simulink model "quadrotor_control_template_R2018a"  (R2021a)
settings: Solver=VariableStepAuto  StartTime=0.0  StopTime=30  MaxStep=0.001  RelTol=1e-6
PreLoadFcn:
  | % first load parameters
  | initializeQuadrotorModel;
values from neighbouring files (symbols this model uses):
  xd0 = [1,2,5]+randn(1,3)    [Project.m]
undefined symbols (not defined in the file or in its folder): quadrotor, simPar
libraries: simulink x4, sharedtransform x1
settings Model: Creator=beniamino  LastModifiedBy=pasqu
settings SolverCC: ZeroCrossAlgorithm=Adaptive  AlgebraicLoopSolver=TrustRegion
settings DebuggingCC: IgnoredZcDiagnostic=none  ArithmeticOperatorsInVariantConditions=warning
settings SFSimCC: CustomCodeUndefinedFunction=UseInterfaceOnly

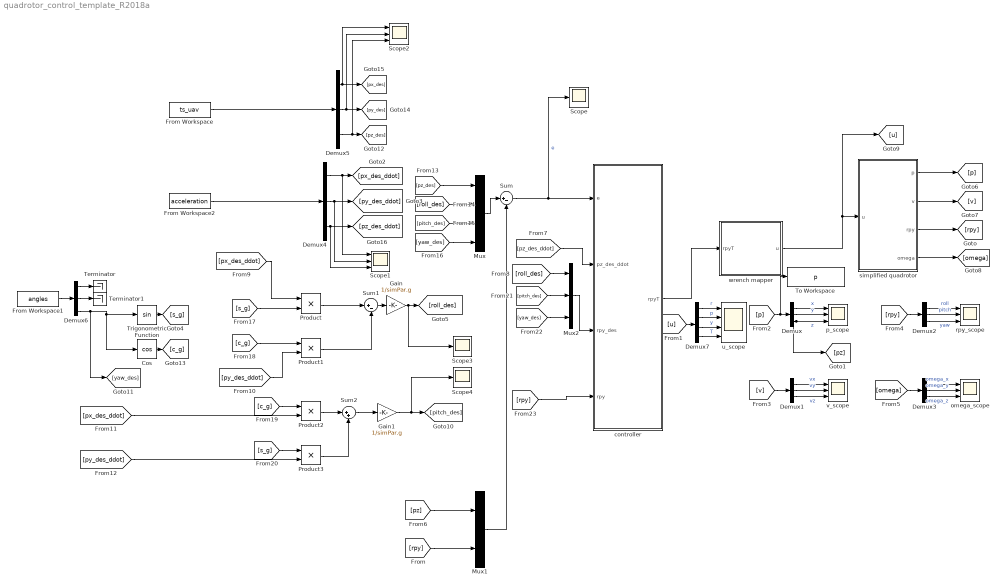
== system quadrotor_control_template_R2018a ==
  Cos : Trigonometry  Operator=cos
  Demux{,1..6} (7 alike) : Demux  Outputs=3
  Demux7 : Demux
  From Workspace : FromWorkspace  VariableName=ts_uav  SampleTime=-1
  From Workspace1 : FromWorkspace  VariableName=angles  SampleTime=-1  OutputAfterFinalValue=Holding final value
  From Workspace2 : FromWorkspace  VariableName=acceleration  SampleTime=-1
  Gain : Gain  Gain=1/simPar.g
  Gain1 : Gain  Gain=1/simPar.g
  Mux : Mux
  Mux1 : Mux  Inputs=2
  Mux2 : Mux  Inputs=3
  Product{,1..3} (4 alike) : Product
  Scope : Scope
  Scope1 : Scope  NumInputPorts=3
  Scope2 : Scope  NumInputPorts=3
  Scope3 : Scope
  Scope4 : Scope
  Sum : Sum  Inputs=|+-
  Sum1 : Sum  Inputs=|+-
  Sum2 : Sum  Inputs=|++
  Terminator : Terminator
  Terminator1 : Terminator
  To Workspace : ToWorkspace  VariableName=p  SaveFormat=Structure With Time  SampleTime=-1
  Trigonometric Function : Trigonometry
  controller : Subsystem
  omega_scope : Scope  NumInputPorts=3
  p_scope : Scope  NumInputPorts=3
  rpy_scope : Scope  NumInputPorts=3
  simplified quadrotor : Subsystem  mask(quadrotor model){F=quadrotor.mixer.F, M=quadrotor.mixer.M, mass=quadrotor.geometry.mass, gravity=simPar.g, inertia=quadrotor.geometry.I, maxRotorSpeed2=quadrotor.rotor.maxRotVelocity.^2, minRotorSpeed2=0, v_0=[0 0 0], omega_0=[0 0 0], ang_0=[0 0 0], p_0=xd0}
      mask prompts: F "F matrix"; M "M matrix"; mass "quadrotor mass"; inertia "inertia matrix"; maxRotorSpeed2 "Rotor max speed square"; minRotorSpeed2 "Rotor min speed square"; v_0 "initial linear velocity"; omega_0 "initial angular velocity"; ang_0 "initial angle"; p_0 "initial position"
      mask help: small angle simplified quadrotor model
      mask TypeOptions F: u2F/Gain
      mask TypeOptions M: u2M/Gain
      mask TypeOptions mass: mass/Value
      mask TypeOptions gravity: small angles rigid body dynamics/gravity/Value
      mask TypeOptions inertia: inertia/Value
      mask TypeOptions maxRotorSpeed2: saturate input/UpperLimit
      mask TypeOptions minRotorSpeed2: saturate input/LowerLimit
      mask TypeOptions v_0: small angles rigid body dynamics/ddp2dp/InitialCondition
      mask TypeOptions omega_0: small angles rigid body dynamics/domega2omega/InitialCondition
      mask TypeOptions ang_0: small angles rigid body dynamics/omega2ang/InitialCondition
      mask TypeOptions p_0: small angles rigid body dynamics/dp2p/InitialCondition
      mask DialogControl InitialConditionsGroupVar Prompt: Initial conditions
  u_scope : Scope  NumInputPorts=4
  v_scope : Scope  NumInputPorts=3
  wrench mapper : Subsystem  mask(wrench mapper){mapperMatrix=quadrotor.mixer.wrenchMapper}
      mask prompts: mapperMatrix "mapper matrix"
      mask help:
      | maps desired roll, pitch, yaw torque and total common thrust into the input vector u for a quadrotor.
      | input: [tau_roll, tau_pitch, tau_yaw, thrust]
      | input unit: [Nm, Nm, Nm, N]
      | output [u_1, u_2, u_3, u_3]
      | output unit: [rad^2/s^2]
      mask TypeOptions mapperMatrix: mapper/Gain
  wires:
  wrench mapper/1(u) -> [u], simplified quadrotor/1(u)
  simplified quadrotor/3(rpy) -> [rpy]
  simplified quadrotor/1(p) -> [p]
  simplified quadrotor/2(v) -> [v]
  simplified quadrotor/4(omega) -> [omega]
  Sum/1 -> Scope/1, controller/1(e)  "e"
  controller/1(rpyT) -> wrench mapper/1(rpyT)
  [p] -> To Workspace/1, Demux/1
  Demux/1 -> p_scope/1  "x"
  Demux/2 -> p_scope/2  "y"
  Demux/3 -> p_scope/3, [pz]  "z"
  [v] -> Demux1/1
  Demux1/2 -> v_scope/2  "vy"
  Demux1/3 -> v_scope/3  "vz"
  Demux1/1 -> v_scope/1  "vx"
  [rpy] -> Demux2/1
  Demux2/2 -> rpy_scope/2  "pitch"
  Demux2/3 -> rpy_scope/3  "yaw"
  Demux2/1 -> rpy_scope/1  "roll"
  [omega] -> Demux3/1
  Demux3/2 -> omega_scope/2  "omega_y"
  Demux3/3 -> omega_scope/3  "omega_z"
  Demux3/1 -> omega_scope/1  "omega_x"
  Mux/1 -> Sum/1
  [rpy] -> Mux1/2
  [pz] -> Mux1/1
  Mux1/1 -> Sum/2
  [pz_des_ddot] -> controller/2(pz_des_ddot)
  Mux2/1 -> controller/3(rpy_des)
  Demux4/1 -> Scope1/1, [px_des_ddot]
  Demux4/2 -> Scope1/2, [py_des_ddot]
  Demux4/3 -> Scope1/3, [pz_des_ddot]
  [px_des_ddot] -> Product/1
  [py_des_ddot] -> Product1/2
  Product/1 -> Sum1/1
  Product1/1 -> Sum1/2
  Sum1/1 -> Gain/1
  Gain/1 -> Scope3/1, [roll_des]
  [px_des_ddot] -> Product2/2
  [py_des_ddot] -> Product3/2
  Product2/1 -> Sum2/1
  Product3/1 -> Sum2/2
  Sum2/1 -> Gain1/1
  Gain1/1 -> Scope4/1, [pitch_des]
  Demux5/3 -> Scope2/3, [pz_des]
  Demux5/2 -> Scope2/2, [py_des]
  Demux5/1 -> Scope2/1, [px_des]
  [roll_des] -> Mux/2
  [pitch_des] -> Mux/3
  [yaw_des] -> Mux/4
  Trigonometric Function/1 -> [s_g]
  Cos/1 -> [c_g]
  [s_g] -> Product/2
  [c_g] -> Product1/1
  [c_g] -> Product2/1
  [s_g] -> Product3/1
  [pz_des] -> Mux/1
  [roll_des] -> Mux2/1
  [pitch_des] -> Mux2/2
  [yaw_des] -> Mux2/3
  [rpy] -> controller/4(rpy)
  From Workspace1/1 -> Demux6/1
  Demux6/3 -> Cos/1, Trigonometric Function/1, [yaw_des]
  Demux6/1 -> Terminator/1
  Demux6/2 -> Terminator1/1
  From Workspace/1 -> Demux5/1
  [u] -> Demux7/1
  Demux7/1 -> u_scope/1  "r"
  Demux7/2 -> u_scope/2  "p"
  Demux7/3 -> u_scope/3  "y"
  Demux7/4 -> u_scope/4  "T"
  From Workspace2/1 -> Demux4/1

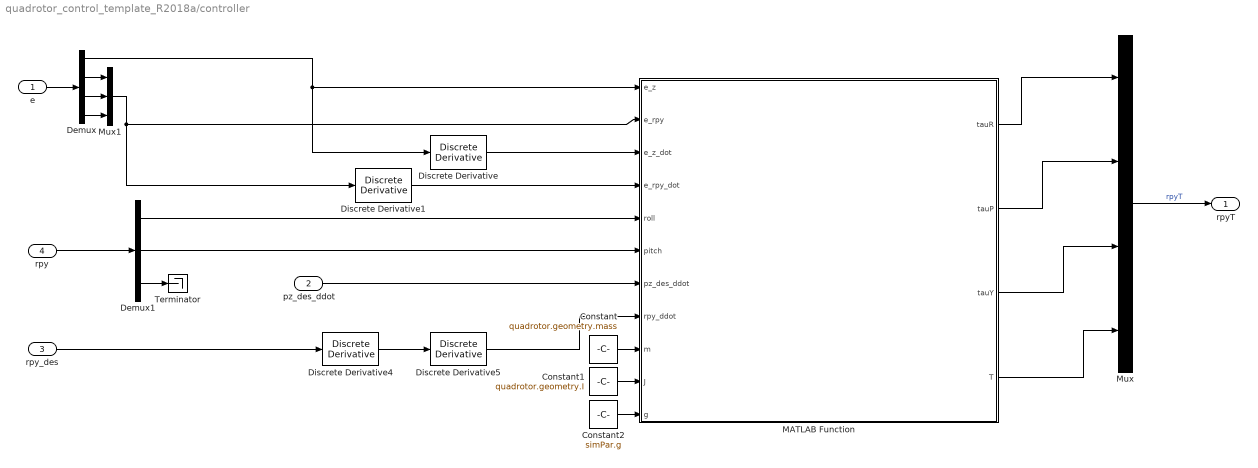
== system quadrotor_control_template_R2018a/controller ==
  e : Inport
  pz_des_ddot : Inport  Port=2
  rpy_des : Inport  Port=3
  rpy : Inport  Port=4
  Constant : Constant  Value=quadrotor.geometry.mass
  Constant1 : Constant  Value=quadrotor.geometry.I
  Constant2 : Constant  Value=simPar.g
  Demux : Demux
  Demux1 : Demux  Outputs=3
  Discrete Derivative{,1,4..5} (4 alike) : simulink/Discrete/Discrete Derivative  gainval=1.0  ICPrevScaledInput=0.0  OutMin=[]  OutMax=[]  OutDataType=fixdt(1, 16)  OutScaling=2^-10  DoSatur=off
  MATLAB Function : MATLAB Function  TreatAsAtomicUnit=on
  Mux : Mux
  Mux1 : Mux  Inputs=3
  Terminator : Terminator
  rpyT : Outport
  wires:
  Mux/1 -> rpyT/1  "rpyT"
  Discrete Derivative/1 -> MATLAB Function/3(e_z_dot)
  Discrete Derivative1/1 -> MATLAB Function/4(e_rpy_dot)
  rpy_des/1 -> Discrete Derivative4/1
  Discrete Derivative4/1 -> Discrete Derivative5/1
  Discrete Derivative5/1 -> MATLAB Function/8(rpy_ddot)
  MATLAB Function/1(tauR) -> Mux/1
  MATLAB Function/2(tauP) -> Mux/2
  MATLAB Function/3(tauY) -> Mux/3
  e/1 -> Demux/1
  Demux/1 -> Discrete Derivative/1, MATLAB Function/1(e_z)
  Demux/3 -> Mux1/2
  Demux/2 -> Mux1/1
  Demux/4 -> Mux1/3
  Mux1/1 -> Discrete Derivative1/1, MATLAB Function/2(e_rpy)
  Constant/1 -> MATLAB Function/9(m)
  Constant1/1 -> MATLAB Function/10(J)
  Constant2/1 -> MATLAB Function/11(g)
  MATLAB Function/4(T) -> Mux/4
  pz_des_ddot/1 -> MATLAB Function/7(pz_des_ddot)
  rpy/1 -> Demux1/1
  Demux1/1 -> MATLAB Function/5(roll)
  Demux1/2 -> MATLAB Function/6(pitch)
  Demux1/3 -> Terminator/1

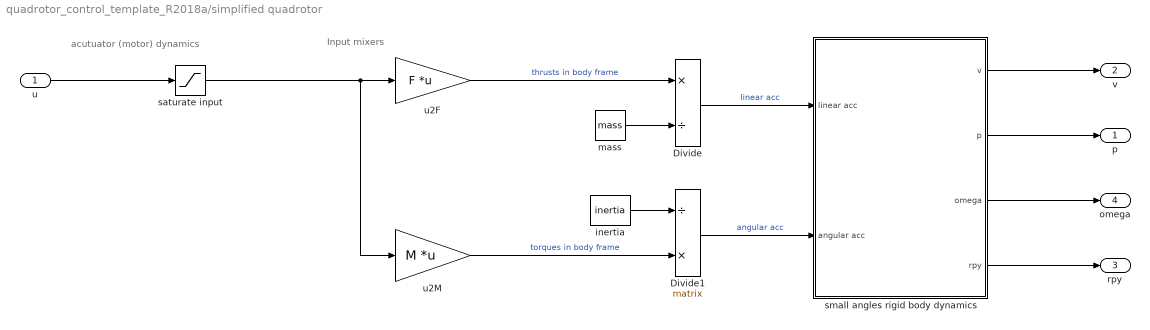
== system quadrotor_control_template_R2018a/simplified quadrotor ==
  note: Input mixers
  note: acutuator (motor) dynamics
  u : Inport
  Divide : Product  Inputs=*/
  Divide1 : Product  Inputs=/*  Multiplication=Matrix(*)
  inertia : Constant  Value=inertia
  mass : Constant  Value=mass
  saturate input : Saturate  UpperLimit=maxRotorSpeed2  LowerLimit=minRotorSpeed2
  small angles rigid body dynamics : Subsystem
  u2F : Gain  Gain=F  Multiplication=Matrix(K*u)
  u2M : Gain  Gain=M  Multiplication=Matrix(K*u)
  p : Outport  PortDimensions=3
  v : Outport  Port=2  PortDimensions=3
  rpy : Outport  Port=3  PortDimensions=3
  omega : Outport  Port=4  PortDimensions=3
  wires:
  small angles rigid body dynamics/4(rpy) -> rpy/1
  small angles rigid body dynamics/3(omega) -> omega/1
  small angles rigid body dynamics/2(p) -> p/1
  small angles rigid body dynamics/1(v) -> v/1
  Divide1/1 -> small angles rigid body dynamics/2(angular acc)  "angular acc"
  Divide/1 -> small angles rigid body dynamics/1(linear acc)  "linear acc"
  u/1 -> saturate input/1
  inertia/1 -> Divide1/1
  u2M/1 -> Divide1/2  "torques in body frame"
  u2F/1 -> Divide/1  "thrusts in body frame"
  mass/1 -> Divide/2
  saturate input/1 -> u2F/1, u2M/1

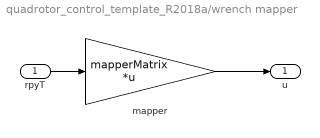
== system quadrotor_control_template_R2018a/wrench mapper ==
  rpyT : Inport
  mapper : Gain  Gain=mapperMatrix  Multiplication=Matrix(K*u)
  u : Outport
  wires:
  mapper/1 -> u/1
  rpyT/1 -> mapper/1

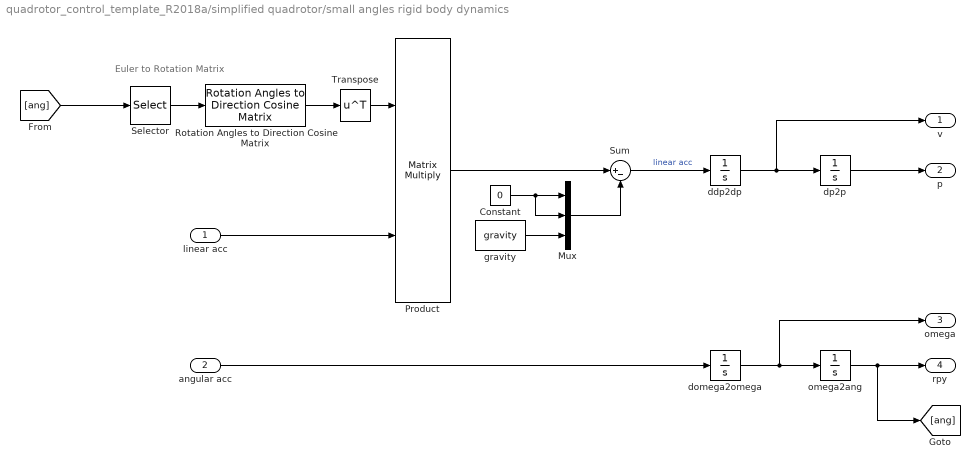
== system quadrotor_control_template_R2018a/simplified quadrotor/small angles rigid body dynamics ==
  note: Euler to Rotation Matrix
  linear acc : Inport
  angular acc : Inport  Port=2
  Constant : Constant  Value=0
  Mux : Mux  Inputs=3
  Product : Product  Multiplication=Matrix(*)
  Rotation Angles to Direction Cosine Matrix : sharedtransform/Rotation Angles to Direction Cosine Matrix  rotationOrder=ZYX  aMode=aMode
      settings: SourceProductBaseCode=AE,PW,DR,MT,UV,VE
  Selector : Selector  InputPortWidth=3  IndexOptions=Index vector (dialog)  Indices=[3 2 1]  OutputSizes=1
  Sum : Sum  Inputs=|+-
  Transpose : Math  Operator=transpose  SignedPower=on  SaturateOnIntegerOverflow=on
  ddp2dp : Integrator  InitialCondition=v_0  ContinuousStateAttributes='v'
  domega2omega : Integrator  InitialCondition=omega_0  ContinuousStateAttributes='omega'
  dp2p : Integrator  InitialCondition=p_0  ContinuousStateAttributes='position'
  gravity : Constant  Value=gravity
  omega2ang : Integrator  InitialCondition=ang_0  ContinuousStateAttributes='rpy'
  v : Outport
  p : Outport  Port=2
  omega : Outport  Port=3
  rpy : Outport  Port=4
  wires:
  Mux/1 -> Sum/2
  [ang] -> Selector/1
  angular acc/1 -> domega2omega/1
  gravity/1 -> Mux/3
  ddp2dp/1 -> dp2p/1, v/1
  linear acc/1 -> Product/2
  Transpose/1 -> Product/1
  Product/1 -> Sum/1
  domega2omega/1 -> omega2ang/1, omega/1
  dp2p/1 -> p/1
  Sum/1 -> ddp2dp/1  "linear acc"
  Constant/1 -> Mux/1, Mux/2
  Selector/1 -> Rotation Angles to Direction Cosine Matrix/1
  omega2ang/1 -> [ang], rpy/1
  Rotation Angles to Direction Cosine Matrix/1 -> Transpose/1

== matlab function quadrotor_control_template_R2018a/controller/MATLAB Function ==
  data: tauR output; tauP output; tauY output; e_z input; e_rpy input; e_z_dot input; e_rpy_dot input; T output; roll input; pitch input; pz_des_ddot input; rpy_ddot input; m input; J input; g input
function [tauR,tauP,tauY,T] = trajectoryQuadrotor(e_z,e_rpy,e_z_dot,e_rpy_dot,roll,pitch,pz_des_ddot,rpy_ddot,m,J,g)
Kp=[100,100,100,100]; %z,r,p,y
Kd=[1,1,1,1]; %z,r,p,y


T=(m/(cos(pitch)*cos(roll)))*(g+pz_des_ddot+Kp(1)*e_z+Kd(1)*e_z_dot);
tauR=J(1,1)*rpy_ddot(1)+Kp(2)*e_rpy(1)+Kd(2)*e_rpy_dot(1);
tauP=J(2,2)*rpy_ddot(2)+Kp(3)*e_rpy(2)+Kd(3)*e_rpy_dot(2);
tauY=J(3,3)*rpy_ddot(3)+Kp(4)*e_rpy(3)+Kd(4)*e_rpy_dot(3);
